simulink model "A9_KGT_Stellantrieb_Kupplung"  (R2017b)
settings: Solver=ode45  StartTime=0.0  StopTime=5  FixedStep=0.00001  MaxStep=1E-4  RelTol=1e-3  EnableMultiTasking=on
values from neighbouring files (symbols this model uses):
  CD = 1e1    (= 10)    [A14_Konstanten.m]    (also in A17_Konstanten.m = 100; A8_Konstanten.m = 20; A9_Konstanten.m = 0.1)
  CF = 1e4    (= 10000)    [A13_Konstanten.m]    (also in A14_Konstanten.m; A17_Konstanten.m = 50000; A8_Konstanten.m = 10000000; A9_Konstanten.m)
  CR = 0.2    [A13_Konstanten.m]    (also in A14_Konstanten.m; A17_Konstanten.m = 100; A9_Konstanten.m = 1; Z_Parametrisierung_Skript.m = [0.5,1,5])
  J2 = (P/(2*pi))^2*m2    (= 0.00283699314199)    [A9_Konstanten.m]
  JK = 1e-4    (= 0.0001)    [A9_Konstanten.m]
  JR = 1.32e-6    (= 1.32e-06)    [A10_Konstanten.m]    (also in A13_Konstanten.m; A14_Konstanten.m; A16_Konstanten.m; A9_Konstanten.m = 0.004)
  P = 0.02    [A8_Konstanten.m]    (also in A9_Konstanten.m = 0.04)
undefined symbols (not defined in the file or in its folder): sigbuilder_block
settings Model: Creator=jbaur  LastModifiedBy=jbaur
settings DataIOCC: ExternalInput=X1  SaveFormat=StructureWithTime  InspectSignalLogs=on  SignalLoggingName=sigsOut
settings OptimizationCC: ExpressionDepthLimit=2147483647  InitFltsAndDblsToZero=on  LifeSpan=inf
settings DebuggingCC: SaveWithParameterizedLinksMsg=none  SignalResolutionControl=TryResolveAllWithWarning  MultiTaskDSMMsg=warning  MultiTaskCondExecSysMsg=none  StateNameClashWarn=warning  SFUnexpectedBacktrackingDiag=warning  SFNoUnconditionalDefaultTransitionDiag=warning  SFExecutionAtInitializationDiag=none
settings HardwareCC: ProdBitPerPointer=32  ProdBitPerSizeT=32  ProdBitPerPtrDiffT=32  ProdLargestAtomicFloat=None  ProdIntDivRoundTo=Undefined  ProdEndianess=Unspecified  ProdWordSize=32  ProdHWDeviceType=32-bit Generic  TargetUnknown=on
settings ModelReferenceCC: PropagateSignalLabelsOutOfModel=off
settings CodeAppCC: StateflowObjectComments=on
settings GRTTargetCC: TargetFcnLib=ansi_tfl_tmw.mat  TargetLangStandard=C89/C90 (ANSI)  ModelReferenceCompliant=off  GeneratePreprocessorConditionals=Disable all  CombineOutputUpdateFcns=off  MatFileLogging=off  GRTInterface=on
settings ConfigComp: CovMetricSettings=dw  CovHtmlReporting=on  CovSaveCumulativeToWorkspaceVar=on  CovSaveSingleToWorkspaceVar=on  CovExternalEMLEnable=off  CovSFcnEnable=off

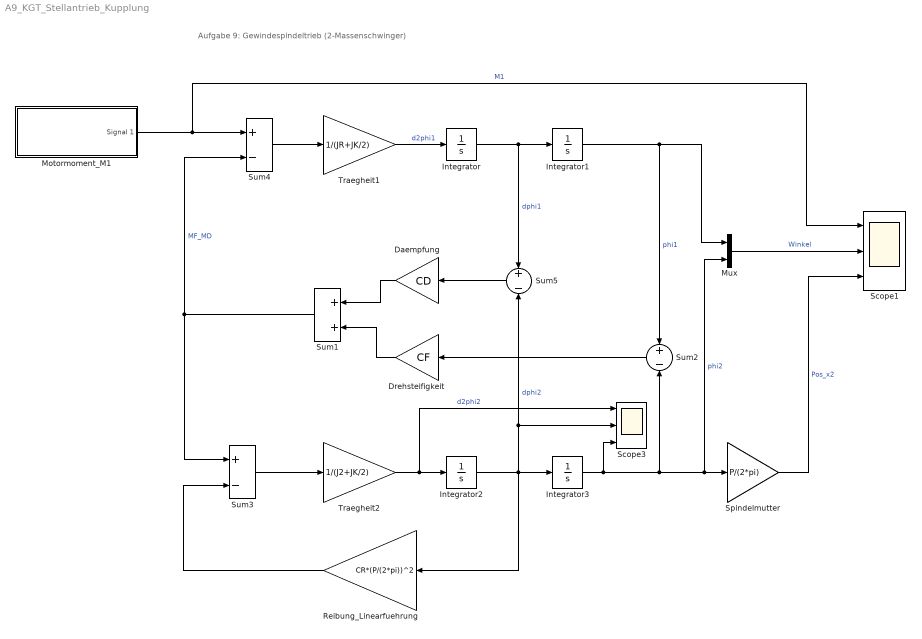
== system A9_KGT_Stellantrieb_Kupplung ==
  note: Aufgabe 9: Gewindespindeltrieb (2-Massenschwinger)
  Daempfung : Gain  Gain=CD
  Drehsteifigkeit : Gain  Gain=CF
  Integrator{,1..3} (4 alike) : Integrator
  Motormoment_M1 : Subsystem  Tag=STV Subsys  LoadFcn=sigbuilder_block('load');  StartFcn=sigbuilder_block('start');  StopFcn=sigbuilder_block('stop');  ClipboardFcn=sigbuilder_block('clipboard');  mask(Sigbuilder block){tuvar=[0:10]}
      mask help: Sigbuilder GUI
      mask init:
      | if ~strcmp(get_param(bdroot(gcbh),'SimulationStatus'),'stopped') tuvar = sigbuilder_block('maskInit'); end
      settings: CopyFcn=sigbuilder_block('copy');  DeleteFcn=sigbuilder_block('delete');  ModelCloseFcn=sigbuilder_block('modelClose');  PreSaveFcn=sigbuilder_block('preSave');  PauseFcn=sigbuilder_block('pause')  ContinueFcn=sigbuilder_block('continue')  NameChangeFcn=sigbuilder_block('namechange');  OpenFcn=sigbuilder_block('open',[49.5 50.25 519.75 399.75 ]);  CloseFcn=sigbuilder_block('close');
      mask Display: plot(0, 0, 100, 100,[2, 2, 32, 32, 2], [68, 8, 8, 68, 68],[32, 2], [38, 38], [32, 19, 2],[53, 60, 44], [32, 17, 17, 2],[16, 16, 31, 31]);txt = getActiveGroup(gcbh);text(2, 100, txt,'verticalAlignment', 'top');
  Mux : Mux  Inputs=2
  Reibung_Linearfuehrung : Gain  Gain=CR*(P/(2*pi))^2
  Scope1 : Scope  NumInputPorts=3
  Scope3 : Scope  NumInputPorts=3
  Spindelmutter : Gain  Gain=P/(2*pi)
  Sum1 : Sum
  Sum{2..5} (4 alike) : Sum  Inputs=+-
  Traegheit1 : Gain  Gain=1/(JR+JK/2)
  Traegheit2 : Gain  Gain=1/(J2+JK/2)
  wires:
  Motormoment_M1/1(Signal 1) -> Scope1/1, Sum4/1  "M1"
  Traegheit1/1 -> Integrator/1  "d2phi1"
  Integrator/1 -> Sum5/1, Integrator1/1  "dphi1"
  Mux/1 -> Scope1/2  "Winkel"
  Traegheit2/1 -> Integrator2/1, Scope3/1  "d2phi2"
  Integrator2/1 -> Sum5/2, Scope3/2, Integrator3/1, Reibung_Linearfuehrung/1  "dphi2"
  Sum3/1 -> Traegheit2/1
  Integrator3/1 -> Scope3/3, Spindelmutter/1, Mux/2, Sum2/2  "phi2"
  Integrator1/1 -> Sum2/1, Mux/1  "phi1"
  Sum2/1 -> Drehsteifigkeit/1
  Sum4/1 -> Traegheit1/1
  Drehsteifigkeit/1 -> Sum1/2
  Daempfung/1 -> Sum1/1
  Sum5/1 -> Daempfung/1
  Reibung_Linearfuehrung/1 -> Sum3/2
  Sum1/1 -> Sum4/2, Sum3/1  "MF_MD"
  Spindelmutter/1 -> Scope1/3  "Pos_x2"

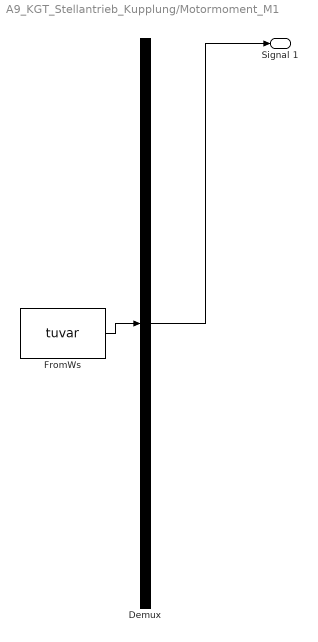
== system A9_KGT_Stellantrieb_Kupplung/Motormoment_M1 ==
  Demux : Demux  Tag=STV Demux  Outputs=1
  FromWs : FromWorkspace  Tag=STV FromWs  VariableName=tuvar  SampleTime=0
      SigBuilderData=|
      | dataSet.timeRange = [0 4]
      | dataSet.name = 'Group 1'
      | sbobj.Groups.Name = 'Group 1'
      | sbobj.Groups.Signals.Name = 'Signal 1'
      | sbobj.Groups.Signals.XData = [0 1 1 2 2 4]
      | sbobj.Groups.Signals.YData = [0 0 10 10 0 0]
      | sbobj.Groups.TimeRange = [0 4]
  Signal 1 : Outport  Tag=STV Outport
  wires:
  Demux/1 -> Signal 1/1
  FromWs/1 -> Demux/1
